simulink model "IM_D03_VFD_5HP"  (R2024a)
settings: Solver=VariableStepAuto  StartTime=0.0  StopTime=1/60  RelTol=1e-3
libraries: simulink x2, spspowerguiLib x1
settings Model: Creator=pc  LastModifiedBy=pc

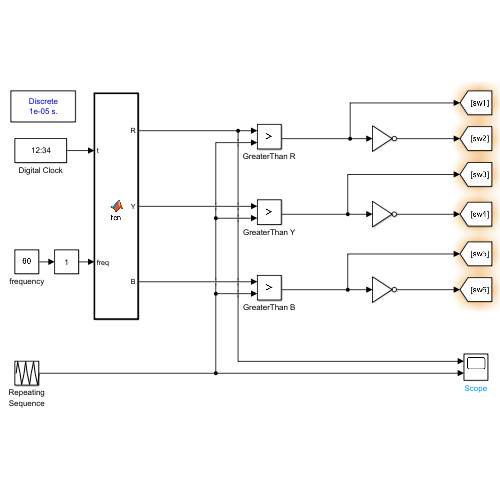
[thumbnail: Simulink's stored preview of the top-level diagram]
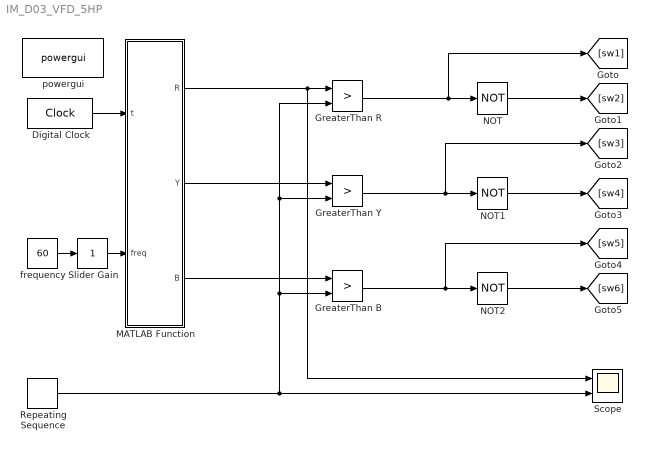
== system IM_D03_VFD_5HP ==
  Digital Clock : DigitalClock  SampleTime=1e-05
  GreaterThan B : RelationalOperator  Operator=>  OutDataTypeStr=boolean  RndMeth=Simplest  InputSameDT=off
  GreaterThan R : RelationalOperator  Operator=>  OutDataTypeStr=boolean  RndMeth=Simplest  InputSameDT=off
  GreaterThan Y : RelationalOperator  Operator=>  OutDataTypeStr=boolean  RndMeth=Simplest  InputSameDT=off
  MATLAB Function : MATLAB Function  TreatAsAtomicUnit=on
  NOT : Logic  Operator=NOT  IconShape=distinctive  AllPortsSameDT=off  OutDataTypeStr=boolean
  NOT1 : Logic  Operator=NOT  IconShape=distinctive  AllPortsSameDT=off  OutDataTypeStr=boolean
  NOT2 : Logic  Operator=NOT  IconShape=distinctive  AllPortsSameDT=off  OutDataTypeStr=boolean
  Repeating Sequence : simulink/Sources/Repeating Sequence  rep_seq_t=[0 0.25 0.5 0.75 1]* (1/5000)  rep_seq_y=[0 1 0 -1 0]
  Scope : Scope  NumInputPorts=2
  Slider Gain : simulink/Math Operations/Slider Gain  gain=1  low=0  high=1
  frequency : Constant  Value=60
  powergui : spspowerguiLib/powergui  Priority=1  SimulationMode=Discrete  SampleTime=1e-05  frequency=60  Iterations=50  frequencyindice=60  Pbase=100e6  ErrMax=1e-4  UnitsV=kV  UnitsW=MW  buscounter=0  FunctionMessages=off  echomessages=off  EnableUseOfTLC=off  CurrentSourceSwitches=off  DisableSnubberDevices=off  DisableRonSwitches=off  DisableVfSwitches=off  DisplayEquations=off  AutomaticDiscreteSolvers=off  SolverType=Tustin/Backward Euler (TBE)  Interpol=off  ExternalGateDelay=off  methode=off  Ts=100  x0status=blocks  SPID=on  SwTol=0  HookPort=off  NonlinearTolerance=1e-4  nMaxIteration=100  ContinueOnMaxIteration=off  RestoreLinks=warning  ResistiveCurrentMeasurement=off  Frange=[0:2:500]  Ylog=off  Xlog=on  ShowGrid=off  save=off  variable=ZData  structure=0  ZoomFFT=off  StartTime=0.0  cycles=1  DisplayStyle=1  fundamental=60  FreqAxis=off  MaxFrequency=1000  frequencyindicesteady=1  RmsSteady=1  display=off
  wires:
  Digital Clock/1 -> MATLAB Function/1(t)
  frequency/1 -> Slider Gain/1
  Slider Gain/1 -> MATLAB Function/2(freq)
  MATLAB Function/2(Y) -> GreaterThan Y/1
  MATLAB Function/1(R) -> Scope/1, GreaterThan R/1
  MATLAB Function/3(B) -> GreaterThan B/1
  Repeating Sequence/1 -> Scope/2, GreaterThan R/2, GreaterThan Y/2, GreaterThan B/2
  GreaterThan R/1 -> [sw1], NOT/1
  GreaterThan Y/1 -> [sw3], NOT1/1
  GreaterThan B/1 -> [sw5], NOT2/1
  NOT/1 -> [sw2]
  NOT1/1 -> [sw4]
  NOT2/1 -> [sw6]

== matlab function IM_D03_VFD_5HP/MATLAB Function ==
  data: t input; R output; freq input; Y output; B output
function [R,Y,B] = fcn(t, freq)
omega = 2*pi*freq;
R = sin(omega*t)*freq/60;
Y = sin(omega*t + 120*pi/180)*freq/60;
B = sin(omega*t + 240*pi/180)*freq/60;
